simulink model "sampleModel1993"  (R2023a)
settings: Solver=VariableStepAuto  StartTime=0.0  StopTime=10.0  RelTol=1e-3
libraries: hdlsllib x3, simulink x2
settings Model: Creator=user1  LastModifiedBy=user1

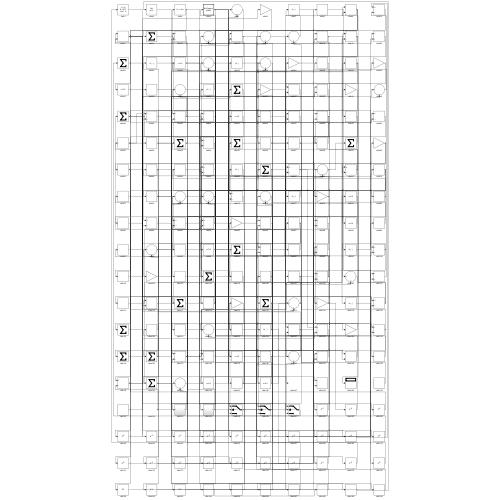
[thumbnail: Simulink's stored preview of the top-level diagram]
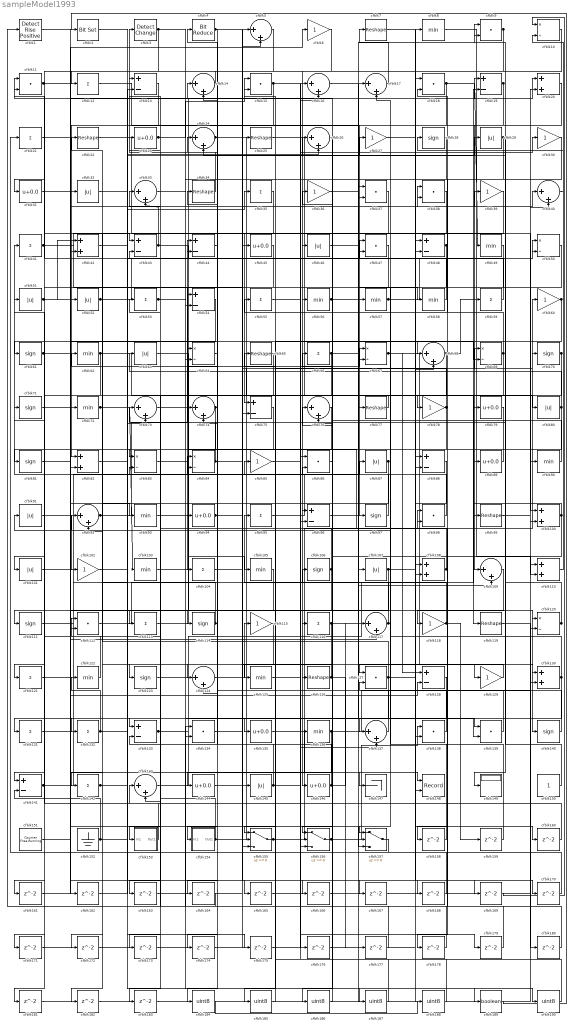
== system sampleModel1993 ==
  cfblk1 : hdlsllib/Logic and Bit Operations/Detect Rise Positive  vinit=0  OutDataTypeStr=boolean
  cfblk{10,50,64,67,69,83..84,120} (8 alike) : Product  Inputs=*/  RndMeth=Zero  SaturateOnIntegerOverflow=on
  cfblk{20,42,82,100,108,110,130} (7 alike) : Sum
  cfblk{29,32,46,51..52,63,80,87,91,101,107,145} (12 alike) : Abs  SaturateOnIntegerOverflow=off
  cfblk{6,27,30,36,39,60,78,85,102,115,118,129} (12 alike) : Gain
  cfblk{8,49,56..58,62,72,90,93,103,105,122,125,136} (14 alike) : MinMax
  cfblk{12,21,35,41,53,55,59,66,95,104,113,116,121,131..132,142} (16 alike) : Sum  Inputs=+
  cfblk{28,61,70..71,81,97,106,111,114,123,140} (11 alike) : Signum
  cfblk{5,14,16..17,24,26,33,40,68,73..74,76,92,109,117,124,137,143} (18 alike) : Sum  Inputs=|++
  cfblk{9,11,15,18,37..38,47,86,98,112,127,134,138..139} (14 alike) : DotProduct  OutDataTypeStr=Inherit: Inherit via internal rule
  cfblk{7,22,25,34,65,77,99,119,126} (9 alike) : Reshape
  cfblk{13,19,43..44,48,54,75,88,96,128,133,141} (12 alike) : Sum  Inputs=+-
  cfblk{23,31,45,79,89,94,135,144,146} (9 alike) : Bias  Bias=0.0  SaturateOnIntegerOverflow=off
  cfblk147 : Terminator
  cfblk148 : Record  FileSettingsInternal="{\"entries\":[{\"content\":{\"excelSettings\":{\"content\":{},\"type\":\"Streamout.ExcelSettings\"}},\"type\":\"Streamout.FileSettingStorage\",\"uuid\":\"\"}],\"packageUris\":[\"http:\\/\\/schema.mathworks.com\\/mf0\\/streamout_blocks\\/R2020a\"],\"version\":\"1.0\"}"  Layout=[1 1]  SignalsInternal="{\"entries\":[{\"content\":{\"signals\":[{\"content\":{\"blockPath\":[],\"dimensions\":[1],\"domain\":\"\",\"lineColor\":\"#a2142f\",\"plots\":[1],\"port\":1,\"signalID\":5720,\"signalName\":\"XY Graph:1\"},\"type\":\"RecordBlkView.Signal\",\"uuid\":\"\"},{\"content\":{\"blockPath\":[],\"dimensions\":[1],\"domain\":\"\",\"lineColor\":\"#139fff\",\"plots\":[1],\"port\":2,\"signalID\":5723,\"signalName\":\"XY Graph:2\"},\"type\":\"RecordBlkView.Signal\",\"uuid\":\"\"}]},\"type\":\"RecordBlkView.InputSignals\",\"uuid\":\"\"}],\"packageUris\":[\"http:\\/\\/schema.mathworks.com\\/mf0\\/streamout_blocks\\/R2020a\"],\"version\":\"1.0\"}"  VisualizationBindings="{\"xyplotplugin\":{\"info\":[{\"series\":[{\"bindingParametersList\":[{\"parameter\":\"X-Axis\",\"signalID\":5720,\"signalName\":\"XY Graph:1\"},{\"parameter\":\"Y-Axis\",\"signalID\":5723,\"signalName\":\"XY Graph:2\"}],\"seriesID\":14439}],\"subplotID\":1}]}}"  CompatibilityTag=XY  st=-1
  cfblk149 : Display
  cfblk150 : Constant  SampleTime=-1
  cfblk151 : hdlsllib/Sources/Counter Free-Running  NumBits=16  tsamp=-1
  cfblk152 : Ground
  cfblk153 : Subsystem
      settings: LibrarySourceBlock=|
      | hdlsllib/Ports &
      | Subsystems/Subsystem
  cfblk154 : Subsystem
      settings: LibrarySourceBlock=|
      | hdlsllib/Ports &
      | Subsystems/Subsystem
  cfblk155 : Switch  SaturateOnIntegerOverflow=off  InputSameDT=off
  cfblk156 : Switch  SaturateOnIntegerOverflow=off  InputSameDT=off
  cfblk157 : Switch  SaturateOnIntegerOverflow=off  InputSameDT=off
  cfblk{158..183} (26 alike) : Delay  SampleTime=1
  cfblk{184..188,190} (6 alike) : DataTypeConversion  OutDataTypeStr=uint8  SaturateOnIntegerOverflow=off  RndMeth=Floor
  cfblk189 : DataTypeConversion  OutDataTypeStr=boolean  SaturateOnIntegerOverflow=off  RndMeth=Floor
  cfblk2 : simulink/Logic and Bit Operations/Bit Set  iBit=0
      settings: LibrarySourceBlock=|
      | hdlsllib/Logic and Bit
      | Operations/Bit Set
  cfblk3 : simulink/Logic and Bit Operations/Detect Change  vinit=0  OutDataTypeStr=boolean
      settings: LibrarySourceBlock=|
      | hdlsllib/Logic and Bit
      | Operations/Detect
      | Change
  cfblk4 : hdlsllib/Logic and Bit Operations/Bit Reduce  mode=AND
  wires:
  cfblk84/1 -> cfblk74/1, cfblk166/1
  cfblk13/1 -> cfblk82/1
  cfblk20/1 -> cfblk97/1
  cfblk140/1 -> cfblk41/1
  cfblk83/1 -> cfblk60/1
  cfblk113/1 -> cfblk20/1
  cfblk151/1 -> cfblk52/1
  cfblk67/1 -> cfblk129/1, cfblk128/1
  cfblk36/1 -> cfblk107/1
  cfblk155/1 -> cfblk98/1, cfblk156/2
  cfblk6/1 -> cfblk146/1
  cfblk130/1 -> cfblk91/1, cfblk141/1
  cfblk72/1 -> cfblk103/1, cfblk27/1
  cfblk41/1 -> cfblk43/1, cfblk145/1
  cfblk3/1 -> cfblk121/1, cfblk187/1
  cfblk154/1(Out1) -> cfblk70/1, cfblk112/1
  cfblk120/1 -> cfblk73/1, cfblk24/2
  cfblk69/1 -> cfblk55/1, cfblk18/2, cfblk178/1
  cfblk110/1 -> cfblk28/1
  cfblk129/1 -> cfblk127/1
  cfblk73/1 -> cfblk67/1
  cfblk90/1 -> cfblk11/1
  cfblk22/1 -> cfblk100/1
  cfblk85/1 -> cfblk30/1
  cfblk141/1 -> cfblk57/1, cfblk128/2
  cfblk81/1 -> cfblk40/1
  cfblk99/1 -> cfblk20/2
  cfblk122/1 -> cfblk71/1
  cfblk117/1 -> cfblk95/1, cfblk157/1
  cfblk92/1 -> cfblk44/1, cfblk35/1
  cfblk124/1 -> cfblk115/1
  cfblk24/1 -> cfblk80/1, cfblk54/1
  cfblk132/1 -> cfblk122/1, cfblk39/1
  cfblk9/1 -> cfblk114/1, cfblk134/2, cfblk174/1
  cfblk156/1 -> cfblk138/1, cfblk106/1
  cfblk60/1 -> cfblk109/1, cfblk155/1
  cfblk37/1 -> cfblk75/1
  cfblk91/1 -> cfblk102/1
  cfblk95/1 -> cfblk87/1
  cfblk108/1 -> cfblk34/1, cfblk84/2
  cfblk114/1 -> cfblk22/1, cfblk64/1
  cfblk96/1 -> cfblk9/1
  cfblk34/1 -> cfblk3/1
  cfblk97/1 -> cfblk23/1
  cfblk8/1 -> cfblk110/2
  cfblk79/1 -> cfblk96/1
  cfblk21/1 -> cfblk93/1
  cfblk19/1 -> cfblk89/1, cfblk112/2
  cfblk144/1 -> cfblk5/1
  cfblk94/1 -> cfblk47/1, cfblk69/1
  cfblk107/1 -> cfblk160/1, cfblk161/1
  cfblk157/1 -> cfblk21/1
  cfblk106/1 -> cfblk33/1, cfblk173/1
  cfblk75/1 -> cfblk81/1
  cfblk12/1 -> cfblk47/2
  cfblk101/1 -> cfblk19/1
  cfblk57/1 -> cfblk50/1, cfblk137/1
  cfblk26/1 -> cfblk116/1
  cfblk38/1 -> cfblk61/1
  cfblk29/1 -> cfblk149/1, cfblk64/2
  cfblk93/1 -> cfblk140/1
  cfblk143/1 -> cfblk45/1
  cfblk47/1 -> cfblk131/1
  cfblk138/1 -> cfblk43/2
  cfblk27/1 -> cfblk18/1
  cfblk25/1 -> cfblk78/1
  cfblk87/1 -> cfblk182/1, cfblk183/1
  cfblk78/1 -> cfblk15/1, cfblk132/1
  cfblk118/1 -> cfblk36/1, cfblk159/1
  cfblk103/1 -> cfblk5/2
  cfblk10/1 -> cfblk154/1(In1)
  cfblk71/1 -> cfblk32/1
  cfblk135/1 -> cfblk148/1
  cfblk66/1 -> cfblk153/1(In1), cfblk69/2
  cfblk54/1 -> cfblk111/1
  cfblk126/1 -> cfblk125/1, cfblk177/1
  cfblk15/1 -> cfblk54/2, cfblk168/1
  cfblk134/1 -> cfblk25/1
  cfblk76/1 -> cfblk133/1
  cfblk33/1 -> cfblk139/1
  cfblk58/1 -> cfblk11/2
  cfblk42/1 -> cfblk26/2
  cfblk89/1 -> cfblk83/1
  cfblk43/1 -> cfblk50/2, cfblk33/2
  cfblk150/1 -> cfblk9/2
  cfblk18/1 -> cfblk49/1, cfblk124/2
  cfblk137/1 -> cfblk62/1
  cfblk63/1 -> cfblk105/1
  cfblk62/1 -> cfblk119/1, cfblk181/1
  cfblk136/1 -> cfblk90/1, cfblk144/1
  cfblk80/1 -> cfblk123/1, cfblk63/1
  cfblk17/1 -> cfblk7/1
  cfblk50/1 -> cfblk77/1
  cfblk1/1 -> cfblk120/1
  cfblk70/1 -> cfblk143/2, cfblk74/2, cfblk92/2
  cfblk152/1 -> cfblk38/1, cfblk141/2
  cfblk145/1 -> cfblk14/1, cfblk16/2, cfblk137/2
  cfblk77/1 -> cfblk72/1
  cfblk123/1 -> cfblk17/1
  cfblk61/1 -> cfblk101/1, cfblk6/1
  cfblk53/1 -> cfblk13/1, cfblk155/3
  cfblk5/1 -> cfblk31/1
  cfblk30/1 -> cfblk118/1
  cfblk121/1 -> cfblk38/2
  cfblk45/1 -> cfblk82/2
  cfblk100/1 -> cfblk99/1, cfblk156/1
  cfblk51/1 -> cfblk147/1, cfblk42/1
  cfblk49/1 -> cfblk104/1
  cfblk4/1 -> cfblk94/1, cfblk130/2, cfblk46/1, cfblk157/2
  cfblk98/1 -> cfblk66/1
  cfblk133/1 -> cfblk19/2, cfblk136/1
  cfblk23/1 -> cfblk15/2, cfblk167/1
  cfblk59/1 -> cfblk4/1
  cfblk88/1 -> cfblk108/2
  cfblk35/1 -> cfblk142/1
  cfblk104/1 -> cfblk29/1
  cfblk153/1(Out1) -> cfblk51/1
  cfblk128/1 -> cfblk135/1
  cfblk116/1 -> cfblk8/1, cfblk124/1
  cfblk39/1 -> cfblk56/1
  cfblk48/1 -> cfblk148/2, cfblk88/2
  cfblk102/1 -> cfblk44/2
  cfblk68/1 -> cfblk126/1, cfblk59/1
  cfblk142/1 -> cfblk84/1, cfblk165/1
  cfblk139/1 -> cfblk17/2
  cfblk64/1 -> cfblk24/1
  cfblk46/1 -> cfblk130/1
  cfblk56/1 -> cfblk58/1, cfblk109/2
  cfblk52/1 -> cfblk16/1, cfblk156/3
  cfblk14/1 -> cfblk12/1
  cfblk40/1 -> cfblk10/2
  cfblk11/1 -> cfblk68/1, cfblk113/1, cfblk117/2, cfblk157/3
  cfblk111/1 -> cfblk13/2
  cfblk74/1 -> cfblk14/2, cfblk163/1
  cfblk28/1 -> cfblk37/1
  cfblk127/1 -> cfblk48/2, cfblk92/1, cfblk185/1
  cfblk112/1 -> cfblk79/1
  cfblk146/1 -> cfblk53/1, cfblk117/1
  cfblk16/1 -> cfblk139/2
  cfblk109/1 -> cfblk158/1
  cfblk158/1 -> cfblk127/2
  cfblk159/1 -> cfblk26/1
  cfblk160/1 -> cfblk143/1
  cfblk161/1 -> cfblk42/2
  cfblk131/1 -> cfblk162/1
  cfblk162/1 -> cfblk73/2
  cfblk163/1 -> cfblk155/2
  cfblk44/1 -> cfblk164/1
  cfblk164/1 -> cfblk1/1
  cfblk165/1 -> cfblk120/2
  cfblk166/1 -> cfblk110/1
  cfblk167/1 -> cfblk100/2
  cfblk168/1 -> cfblk108/1
  cfblk31/1 -> cfblk169/1
  cfblk169/1 -> cfblk10/1
  cfblk7/1 -> cfblk170/1
  cfblk170/1 -> cfblk83/2
  cfblk105/1 -> cfblk171/1
  cfblk171/1 -> cfblk48/1
  cfblk115/1 -> cfblk172/1
  cfblk172/1 -> cfblk138/2
  cfblk173/1 -> cfblk88/1
  cfblk174/1 -> cfblk75/2
  cfblk32/1 -> cfblk175/1
  cfblk175/1 -> cfblk96/2
  cfblk125/1 -> cfblk176/1
  cfblk176/1 -> cfblk67/2
  cfblk177/1 -> cfblk134/1
  cfblk178/1 -> cfblk76/2
  cfblk55/1 -> cfblk179/1
  cfblk179/1 -> cfblk133/2
  cfblk119/1 -> cfblk180/1
  cfblk180/1 -> cfblk98/2
  cfblk181/1 -> cfblk68/2
  cfblk182/1 -> cfblk40/2
  cfblk183/1 -> cfblk37/2
  cfblk65/1 -> cfblk184/1
  cfblk185/1 -> cfblk65/1
  cfblk86/1 -> cfblk186/1
  cfblk186/1 -> cfblk76/1
  cfblk187/1 -> cfblk86/1
  cfblk184/1 -> cfblk188/1
  cfblk188/1 -> cfblk86/2
  cfblk82/1 -> cfblk189/1
  cfblk189/1 -> cfblk2/1
  cfblk2/1 -> cfblk190/1
  cfblk190/1 -> cfblk85/1

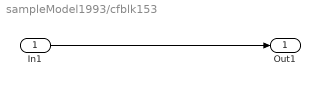
== system sampleModel1993/cfblk153 ==
  In1 : Inport
  Out1 : Outport
  wires:
  In1/1 -> Out1/1

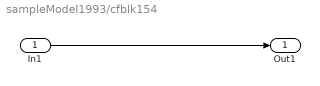
== system sampleModel1993/cfblk154 ==
  In1 : Inport
  Out1 : Outport
  wires:
  In1/1 -> Out1/1
